simulink model "Pendulum_3"  (R2019b)
settings: Solver=VariableStepAuto  StartTime=0.0  StopTime=t_end  MaxStep=t_Max_step  RelTol=1e-3
values from neighbouring files (symbols this model uses):
  C_fv = 0.2    [Pendulumn_1.m]
  g = 9.8    [Pendulumn_1.m]
  L = 0.3    [Pendulumn_1.m]    (also in RLC_S.m = 1)
  m = 0.5    [Pendulumn_1.m]
  omega0 = 5    [Pendulumn_1.m]
  theta0 = 30    [Pendulumn_1.m]
settings Model: Creator=raobo  LastModifiedBy=raobo

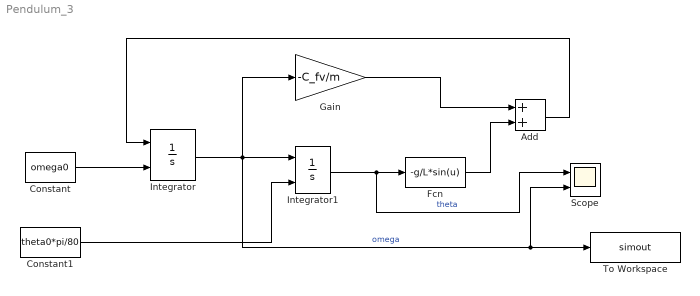
== system Pendulum_3 ==
  Add : Sum
  Constant : Constant  Value=omega0
  Constant1 : Constant  Value=theta0*pi/80
  Fcn : Fcn  Expr=-g/L*sin(u)
  Gain : Gain  Gain=-C_fv/m
  Integrator : Integrator  InitialConditionSource=external
  Integrator1 : Integrator  InitialConditionSource=external
  Scope : Scope  NumInputPorts=2
  To Workspace : ToWorkspace  VariableName=simout  SaveFormat=Timeseries  SampleTime=-1
  wires:
  Integrator/1 -> Gain/1, To Workspace/1, Scope/2, Integrator1/1  "omega"
  Integrator1/1 -> Scope/1, Fcn/1  "theta"
  Constant/1 -> Integrator/2
  Constant1/1 -> Integrator1/2
  Gain/1 -> Add/1
  Fcn/1 -> Add/2
  Add/1 -> Integrator/1
